simulink subsystem "computeLPinv"  (R2020b)
settings: Solver=VariableStepAuto  StartTime=0.0  StopTime=10.0  RelTol=1e-3
settings Model: Creator=marco  LastModifiedBy=marco

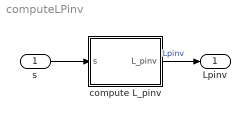
== system computeLPinv ==
  s : Inport
  compute L_pinv : MATLAB Function  TreatAsAtomicUnit=on
  Lpinv : Outport
  wires:
  s/1 -> compute L_pinv/1(s)
  compute L_pinv/1(L_pinv) -> Lpinv/1  "Lpinv"

== matlab function computeLPinv/compute L_pinv ==
  data: s input; L_pinv output
function L_pinv = fcn(s)

L_pinv = computeLpinv(s);
